simulink model "Integration"  (R2024b)
settings: Solver=VariableStepAuto  StartTime=0.0  StopTime=4  RelTol=1e-3
undefined symbols (not defined in the file): Ion, Lithium, Ts_Control
libraries: spsSeriesRLCBranchLib x37, ee_lib x30, nesl_utility x30, spsCurrentVoltageSimscapeInterfaceLib x18, slpidlib x9, spsThreePhaseVIMeasurementLib x7, spsParallelRLCBranchLib x7, spsThreePhaseSeriesRLCBranchLib x7, spsGroundLib x7, spsDiodeLib x6, spsIGBTDiodeLib x6, spsPWMGeneratorDCDCLib x6
(part 1 of 4)
settings Model: Creator=DELL  LastModifiedBy=DELL

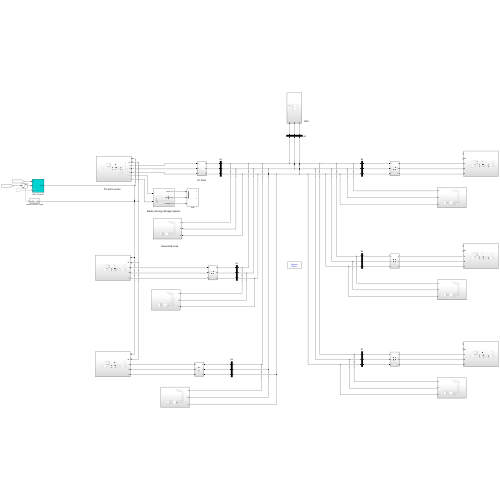
[thumbnail: Simulink's stored preview of the top-level diagram]
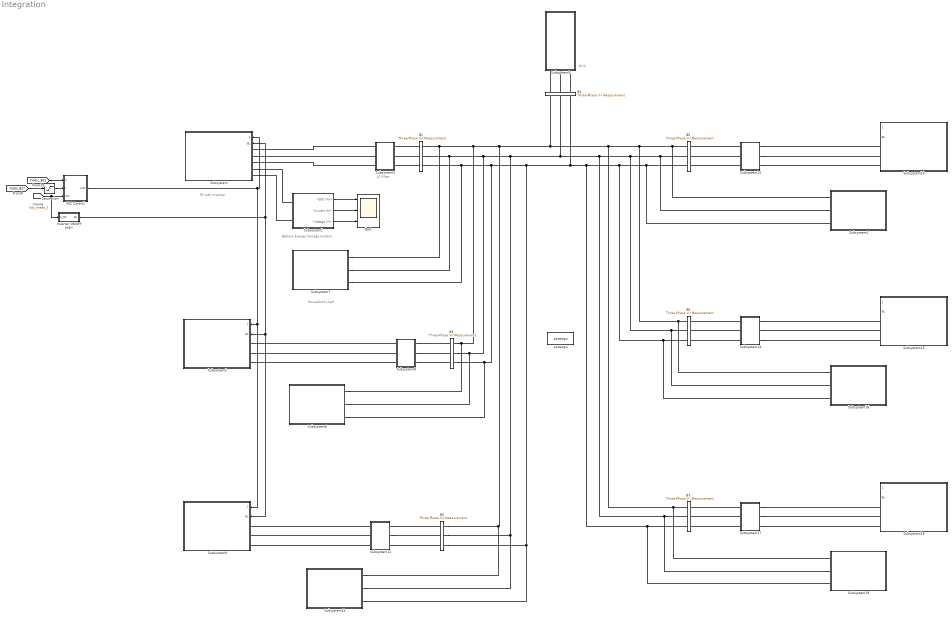
== system Integration ==
  note: Household Load
  note: LC Filter
  note: Battery Energy Storage System
  note: Grid
  note: PV with Inverter
  B1 : spsThreePhaseVIMeasurementLib/Three-Phase V-I Measurement  VoltageMeasurement=phase-to-phase  SetLabelV=on  LabelV=Vabc_B1  Vpu=off  VpuLL=off  CurrentMeasurement=yes  SetLabelI=on  LabelI=Iabc_B1  Ipu=off  Pbase=100e6  Vbase=1000  OutputType=Magnitude  PhasorSimulation=off  PSBequivalent=0
  B2 : spsThreePhaseVIMeasurementLib/Three-Phase V-I Measurement  VoltageMeasurement=phase-to-phase  SetLabelV=on  LabelV=Vabc_B2  Vpu=off  VpuLL=off  CurrentMeasurement=yes  SetLabelI=on  LabelI=Iabc_B2  Ipu=off  Pbase=100e6  Vbase=500e3  OutputType=Magnitude  PhasorSimulation=off  PSBequivalent=0
  B3 : spsThreePhaseVIMeasurementLib/Three-Phase V-I Measurement  VoltageMeasurement=phase-to-phase  SetLabelV=on  LabelV=Vabc_B3  Vpu=off  VpuLL=off  CurrentMeasurement=yes  SetLabelI=on  LabelI=Iabc_B3  Ipu=off  Pbase=100e6  Vbase=1000  OutputType=Magnitude  PhasorSimulation=off  PSBequivalent=0
  B4 : spsThreePhaseVIMeasurementLib/Three-Phase V-I Measurement  VoltageMeasurement=phase-to-phase  SetLabelV=on  LabelV=Vabc_B4  Vpu=off  VpuLL=off  CurrentMeasurement=yes  SetLabelI=on  LabelI=Iabc_B4  Ipu=off  Pbase=100e6  Vbase=1000  OutputType=Magnitude  PhasorSimulation=off  PSBequivalent=0
  B5 : spsThreePhaseVIMeasurementLib/Three-Phase V-I Measurement  VoltageMeasurement=phase-to-phase  SetLabelV=on  LabelV=Vabc_B5  Vpu=off  VpuLL=off  CurrentMeasurement=yes  SetLabelI=on  LabelI=Iabc_B5  Ipu=off  Pbase=100e6  Vbase=1000  OutputType=Magnitude  PhasorSimulation=off  PSBequivalent=0
  B6 : spsThreePhaseVIMeasurementLib/Three-Phase V-I Measurement  VoltageMeasurement=phase-to-phase  SetLabelV=on  LabelV=Vabc_B6  Vpu=off  VpuLL=off  CurrentMeasurement=yes  SetLabelI=on  LabelI=Iabc_B6  Ipu=off  Pbase=100e6  Vbase=1000  OutputType=Magnitude  PhasorSimulation=off  PSBequivalent=0
  B7 : spsThreePhaseVIMeasurementLib/Three-Phase V-I Measurement  VoltageMeasurement=phase-to-phase  SetLabelV=on  LabelV=Vabc_B7  Vpu=off  VpuLL=off  CurrentMeasurement=yes  SetLabelI=on  LabelI=Iabc_B7  Ipu=off  Pbase=100e6  Vbase=1000  OutputType=Magnitude  PhasorSimulation=off  PSBequivalent=0
  Batt : Scope  NumInputPorts=3
  Inverter ON/OFF Logic : Subsystem
  Saturation : Saturate  UpperLimit=40  LowerLimit=-40
  Subsystem : Subsystem
  Subsystem1 : Subsystem
  Subsystem10 : Subsystem
  Subsystem11 : Subsystem
  Subsystem12 : Subsystem
  Subsystem13 : Subsystem
  Subsystem14 : Subsystem
  Subsystem15 : Subsystem
  Subsystem16 : Subsystem
  Subsystem17 : Subsystem
  Subsystem18 : Subsystem
  Subsystem19 : Subsystem
  Subsystem2 : Subsystem
  Subsystem3 : Subsystem
  Subsystem4 : Subsystem
  Subsystem5 : Subsystem
  Subsystem6 : Subsystem
  Subsystem7 : Subsystem
  Subsystem8 : Subsystem
  Subsystem9 : Subsystem
  VSC Control : Subsystem  mask(VSC Main Controller){nom=[ 20e3  50 ], Vnom=[ 400 400 ], Vnom_dc=700, RLxfo=[0  0 ], RLchoke=[0  0  ], K_VDCreg=[18  600], K_Ireg=[0.2 20], Ts=Ts_Control}
      mask prompts: nom "Nominal power and frequency [ Pnom(VA)  Fnom(Hz) ]:"; Vnom "Nominal primary and secondary voltages (Vrms LL) [ Vnom_prim   Vnom_sec ]:"; Vnom_dc "Nominal DC bus voltage (V):"; RLxfo "Total transformer leakage impedance (pu/Pnom) [ Rxfo  Lxf ]"; RLchoke "Choke impedance [ R(ohm) L(H) ]"; K_VDCreg "VDC regultator gains [ Kp  Ki ]:"; K_Ireg "Current regulator gains [ Kp  Ki ]:"; Ts "Sample time"
      mask init:
      | Pnom=nom(1);
      | Fnom=nom(2);
      | Vnom_prim=Vnom(1);
      | Vnom_sec=Vnom(2);
      | Zbase=Vnom_sec^2/Pnom;
      | Rtot_pu=RLxfo(1) + RLchoke(1)/Zbase;
      | Ltot_pu=RLxfo(2) + RLchoke(2)/(Zbase/(2*pi*Fnom));
      | Kp_VDCreg=K_VDCreg(1);
      | Ki_VDCreg=K_VDCreg(2);
      | Kp_Ireg=K_Ireg(1);
      | Ki_Ireg=K_Ireg(2);
      | Vdc_ref=Vnom_dc;
  powergui : spspowerguiLib/powergui  Priority=1  SimulationMode=Discrete  SampleTime=1e-4  frequency=60  Iterations=50  frequencyindice=0  Pbase=100e6  ErrMax=1e-4  UnitsV=kV  UnitsW=MW  buscounter=0  FunctionMessages=off  echomessages=off  EnableUseOfTLC=off  CurrentSourceSwitches=off  DisableSnubberDevices=off  DisableRonSwitches=off  DisableVfSwitches=off  DisplayEquations=off  AutomaticDiscreteSolvers=off  SolverType=Tustin/Backward Euler (TBE)  Interpol=off  ExternalGateDelay=off  methode=off  Ts=100  x0status=blocks  SPID=on  SwTol=0  HookPort=off  NonlinearTolerance=1e-4  nMaxIteration=100  ContinueOnMaxIteration=off  RestoreLinks=warning  ResistiveCurrentMeasurement=off  Frange=[0:2:500]  Ylog=off  Xlog=on  ShowGrid=off  save=off  variable=ZData  structure=0  ZoomFFT=off  StartTime=0.0  cycles=1  DisplayStyle=1  fundamental=60  FreqAxis=off  MaxFrequency=1000  frequencyindicesteady=1  RmsSteady=1  display=off
  wires:
  [Vdc_meas_1] -> Inverter ON/OFF Logic/1(V_DC), VSC Control/3(Vdc)
  [Vabc_B2] -> VSC Control/1(V)
  Saturation/1 -> VSC Control/2(I)
  [Iabc_B2] -> Saturation/1
  Inverter ON/OFF Logic/1(BL) -> Subsystem9/2(BL), Subsystem2/2(BL), Subsystem/2(BL)
  VSC Control/1(Uref) -> Subsystem9/1("  "), Subsystem2/1("  "), Subsystem/1("  ")
  Subsystem1/1(<SOC (%)>) -> Batt/1
  Subsystem1/2(<Current (A)>) -> Batt/2
  Subsystem1/3(<Voltage (V)>) -> Batt/3
  connections:
  B1/RConn1 -- Subsystem7/LConn1 -- Subsystem6/LConn1 -- B3/RConn1 -- Subsystem11/LConn1 -- B4/RConn1 -- Subsystem19/LConn1 -- B7/RConn1 -- Subsystem16/LConn1 -- B6/RConn1 -- Subsystem4/LConn1 -- B5/RConn1 -- B2/RConn1
  B2/RConn3 -- Subsystem11/LConn3 -- B4/RConn3 -- Subsystem6/LConn3 -- B3/RConn3 -- Subsystem7/LConn3 -- B1/RConn3 -- Subsystem19/LConn3 -- B7/RConn3 -- Subsystem16/LConn3 -- B6/RConn3 -- Subsystem4/LConn3 -- B5/RConn3
  B1/RConn2 -- Subsystem7/LConn2 -- Subsystem6/LConn2 -- B3/RConn2 -- Subsystem11/LConn2 -- B4/RConn2 -- Subsystem19/LConn2 -- B7/RConn2 -- Subsystem16/LConn2 -- B6/RConn2 -- Subsystem4/LConn2 -- B5/RConn2 -- B2/RConn2
  B1/LConn3 -- Subsystem3/RConn3
  B1/LConn1 -- Subsystem3/RConn1
  B1/LConn2 -- Subsystem3/RConn2
  Subsystem3/LConn1 -- Subsystem/LConn1
  Subsystem3/LConn2 -- Subsystem/LConn2
  Subsystem3/LConn3 -- Subsystem/LConn3
  B2/LConn1 -- Subsystem5/LConn1
  B2/LConn2 -- Subsystem5/LConn2
  B2/LConn3 -- Subsystem5/LConn3
  Subsystem1/LConn1 -- Subsystem/LConn4
  Subsystem1/LConn2 -- Subsystem/LConn5
  Subsystem8/LConn1 -- Subsystem2/LConn1
  Subsystem8/LConn2 -- Subsystem2/LConn2
  Subsystem8/LConn3 -- Subsystem2/LConn3
  Subsystem8/RConn1 -- B3/LConn1
  Subsystem8/RConn2 -- B3/LConn2
  Subsystem8/RConn3 -- B3/LConn3
  Subsystem12/RConn1 -- B4/LConn1
  Subsystem12/LConn2 -- Subsystem9/LConn2
  Subsystem12/RConn3 -- B4/LConn3
  Subsystem12/LConn3 -- Subsystem9/LConn3
  Subsystem12/LConn1 -- Subsystem9/LConn1
  Subsystem12/RConn2 -- B4/LConn2
  Subsystem10/LConn1 -- Subsystem13/LConn1
  Subsystem10/RConn3 -- B5/LConn3
  Subsystem10/RConn1 -- B5/LConn1
  Subsystem10/LConn3 -- Subsystem13/LConn3
  Subsystem10/LConn2 -- Subsystem13/LConn2
  Subsystem10/RConn2 -- B5/LConn2
  Subsystem14/LConn2 -- Subsystem15/LConn2
  Subsystem14/RConn3 -- B6/LConn3
  Subsystem14/LConn1 -- Subsystem15/LConn1
  Subsystem14/LConn3 -- Subsystem15/LConn3
  Subsystem14/RConn1 -- B6/LConn1
  Subsystem14/RConn2 -- B6/LConn2
  Subsystem17/LConn2 -- Subsystem18/LConn2
  Subsystem17/RConn3 -- B7/LConn3
  Subsystem17/LConn1 -- Subsystem18/LConn1
  Subsystem17/LConn3 -- Subsystem18/LConn3
  Subsystem17/RConn1 -- B7/LConn1
  Subsystem17/RConn2 -- B7/LConn2

== system Integration/Inverter ON//OFF Logic ==
  V_DC : Inport
  AND : Logic  Operator=NAND  IconShape=distinctive  AllPortsSameDT=off  OutDataTypeStr=boolean
  Compare To Constant : simulink/Logic and Bit Operations/Compare To Constant  relop=>=  const=200  OutDataTypeStr=boolean
  Constant : Constant
  Data Type Conversion : DataTypeConversion  OutDataTypeStr=double  SaturateOnIntegerOverflow=off  RndMeth=Floor
  BL : Outport
  tag scope: inv_cont_1=global
  wires:
  Data Type Conversion/1 -> [inv_cont_1], BL/1
  V_DC/1 -> Compare To Constant/1
  AND/1 -> Data Type Conversion/1
  Compare To Constant/1 -> AND/1
  Constant/1 -> AND/2

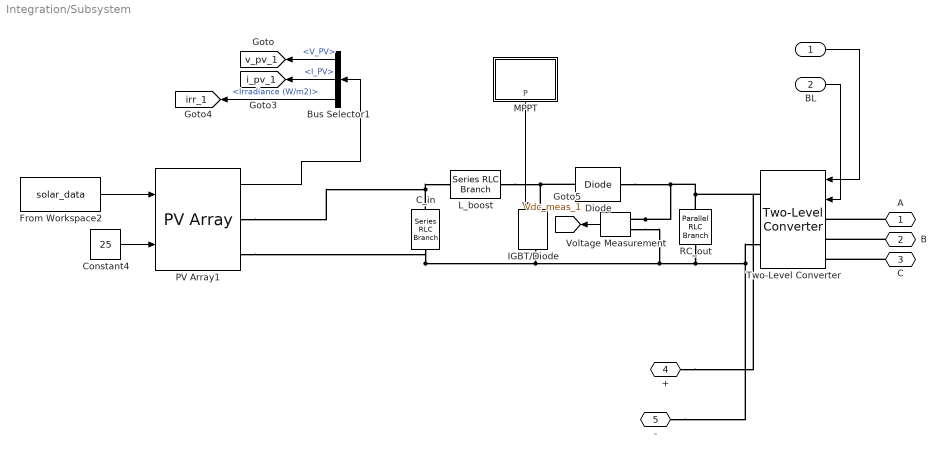
== system Integration/Subsystem ==
  "  " : Inport
  BL : Inport  Port=2
  Bus Selector1 : BusSelector  OutputSignals=V_PV,I_PV,Irradiance (W/m2)
  C_in : spsSeriesRLCBranchLib/Series RLC Branch  LConnTagsString=__new0  RConnTagsString=__new0  BranchType=C  Resistance=1e-5  Inductance=1e-3  SetiL0=off  InitialCurrent=0  Capacitance=850e-6  Setx0=off  InitialVoltage=426.5  Measurements=Branch voltage and current
  Constant4 : Constant  Value=25
  Diode : spsDiodeLib/Diode  Ron=0.001  Lon=0  Vf=0.8  IC=0  UseSnubber=0  Rs=500  Cs=250e-9  Measurements=off
  From Workspace2 : FromWorkspace  VariableName=solar_data  OutDataTypeStr=double  SampleTime=0.01
  IGBT/Diode : spsIGBTDiodeLib/IGBT//Diode  Ron=1e-3  Rs=1e5  Cs=inf  Measurements=off
  L_boost : spsSeriesRLCBranchLib/Series RLC Branch  LConnTagsString=__new0  RConnTagsString=__new0  BranchType=L  Resistance=1e-3  Inductance=36e-3  SetiL0=off  InitialCurrent=0  Capacitance=100e-6  Setx0=off  InitialVoltage=230  Measurements=None
  MPPT : Subsystem
  PV Array1 : spsPVArrayLib/PV Array  Npar=8  Nser=5  PlotType=array @ 1000 W/m2 & specified temperatures  S_vec="[ 1000  500  100 ]"  Temp_C_vec="[ 45 25  ]"  ModuleName=SunPower SPR-415E-WHT-D  PlotWhenSelected=off  Pm=414.801  Ncell=128  Voc=85.3  Isc=6.09  Vm=72.9  Im=5.69  beta_Voc_pc=-0.229  alpha_Isc_pc=0.030706  beta_Voc=-0.19534  alpha_Isc=0.00187  IL=6.0978  I0=7.1698e-13  nI=0.87223  Rsh=419.7781  Rs=0.53711  RobustModel=off  RobustCellTemperature=313.3991  BAL=on  Tc=1e-6  Tfilter=5e-5
  RC_out : spsParallelRLCBranchLib/Parallel RLC Branch  LConnTagsString=a  RConnTagsString=__new0  BranchType=C  Resistance=5  Inductance=1e-3  SetiL0=off  InitialCurrent=0  Capacitance=5*636e-6  Setx0=off  InitialVoltage=700  Measurements=None
  Two-Level Converter : spsTwoLevelConverterLib/Two-Level Converter  ModelType=Switching devices  Ron=1e-3  Rs=1e6  Cs=inf  Vforward=[0,0]  Ron_Diode=1e-3  Rs_Diode=1e6  Cs_Diode=inf  Vf_Diode=1e-3  Rs_CurrentSource=inf  Ron_ACsource=1e-3
      settings: LibrarySourceBlock=sps_lib/Power Electronics/Two-Level Converter
  Voltage Measurement : spsVoltageMeasurementLib/Voltage Measurement  PhasorSimulation=off  OutputType=Complex  PSBequivalent=0
  A : PMIOPort  Side=Left
  B : PMIOPort  Port=2  Side=Left
  C : PMIOPort  Port=3  Side=Left
  + : PMIOPort  Port=4  Side=Left
  - : PMIOPort  Port=5  Side=Left
  tag scope: Vdc_meas_1=global, i_pv_1=global, irr_1=global, v_pv_1=global
  wires:
  Voltage Measurement/1 -> [Vdc_meas_1]
  BL/1 -> Two-Level Converter/2
  Bus Selector1/3 -> [irr_1]  "<Irradiance (W/m2)>"
  Bus Selector1/1 -> [v_pv_1]  "<V_PV>"
  Constant4/1 -> PV Array1/2
  "  "/1 -> Two-Level Converter/1
  Bus Selector1/2 -> [i_pv_1]  "<I_PV>"
  PV Array1/1 -> Bus Selector1/1
  MPPT/1(P) -> IGBT/Diode/1
  From Workspace2/1 -> PV Array1/1
  connections:
  A/RConn1 -- Two-Level Converter/LConn1
  PV Array1/RConn2 -- C_in/RConn1 -- IGBT/Diode/RConn1 -- Voltage Measurement/LConn2 -- RC_out/RConn1 -- -/RConn1 -- Two-Level Converter/RConn2
  IGBT/Diode/LConn1 -- L_boost/RConn1 -- Diode/LConn1
  PV Array1/RConn1 -- L_boost/LConn1 -- C_in/LConn1
  Voltage Measurement/LConn1 -- +/RConn1 -- Two-Level Converter/RConn1 -- RC_out/LConn1 -- Diode/RConn1
  C/RConn1 -- Two-Level Converter/LConn3
  B/RConn1 -- Two-Level Converter/LConn2

== system Integration/Subsystem1 ==
  BATT chg-dshg logic : Subsystem
  Battery : spsBatteryLib/Battery  BatType=Lithium-Ion  NomV=24  NomQ=20  SOC=0  Batt_Tr=0.01  PresetModel=on  MaxQ=20  MinV=18  FullV=27.9357  Dis_rate=8.6957  R=0.012  Normal_OP=18.087  expZone="[25.9293     0.982609]"
  Bus Selector : BusSelector  OutputSignals=SOC (%),Current (A),Voltage (V)
  L_B : spsSeriesRLCBranchLib/Series RLC Branch  LConnTagsString=__new0  RConnTagsString=__new0  BranchType=L  Resistance=1e-3  Inductance=1e-3  SetiL0=off  InitialCurrent=0  Capacitance=100e-6  Setx0=off  InitialVoltage=230  Measurements=None
  RC_B : spsParallelRLCBranchLib/Parallel RLC Branch  LConnTagsString=a  RConnTagsString=__new0  BranchType=C  Resistance=5  Inductance=1e-3  SetiL0=off  InitialCurrent=0  Capacitance=50e-6  Setx0=off  InitialVoltage=700  Measurements=None
  Two-Quadrant DC/DC Converter : spsTwoQuadrantDCDCConverterLib/Two-Quadrant DC//DC Converter  ModelType=Average model (D-controlled)  Ron=1e-3  Rs=1e6  Cs=inf  Vforward=[0,0]  Ron_Diode=1e-3  Rs_Diode=1e6  Cs_Diode=inf  Vf_Diode=1e-3  Rs_CurrentSource=inf  Ron_ACsource=1e-3
  + : PMIOPort  Side=Left
  - : PMIOPort  Port=2  Side=Left
  <SOC (%)> : Outport
  <Current (A)> : Outport  Port=2
  <Voltage (V)> : Outport  Port=3
  wires:
  Battery/1 -> Bus Selector/1
  BATT chg-dshg logic/2(BL) -> Two-Quadrant DC/DC Converter/2
  Bus Selector/3 -> <Voltage (V)>/1, BATT chg-dshg logic/2(V_batt)  "<Voltage (V)>"
  Bus Selector/1 -> <SOC (%)>/1, BATT chg-dshg logic/1(SoC)  "<SOC (%)>"
  BATT chg-dshg logic/1(D) -> Two-Quadrant DC/DC Converter/1
  Bus Selector/2 -> <Current (A)>/1  "<Current (A)>"
  connections:
  RC_B/LConn1 -- +/RConn1 -- Two-Quadrant DC/DC Converter/RConn1
  L_B/LConn1 -- Battery/LConn1
  Battery/LConn2 -- -/RConn1 -- RC_B/RConn1 -- Two-Quadrant DC/DC Converter/RConn2
  L_B/RConn1 -- Two-Quadrant DC/DC Converter/LConn1

== system Integration/Subsystem10 ==
  Series RLC Branch1 : spsSeriesRLCBranchLib/Series RLC Branch  LConnTagsString=__new0  RConnTagsString=__new0  BranchType=RC  Resistance=10  Inductance=1e-3  SetiL0=off  InitialCurrent=0  Capacitance=3*15e-6  Setx0=off  InitialVoltage=0  Measurements=None
  Series RLC Branch2 : spsSeriesRLCBranchLib/Series RLC Branch  LConnTagsString=__new0  RConnTagsString=__new0  BranchType=RC  Resistance=10  Inductance=1e-3  SetiL0=off  InitialCurrent=0  Capacitance=3*15e-6  Setx0=off  InitialVoltage=0  Measurements=None
  Series RLC Branch3 : spsSeriesRLCBranchLib/Series RLC Branch  LConnTagsString=__new0  RConnTagsString=__new0  BranchType=RC  Resistance=10  Inductance=1e-3  SetiL0=off  InitialCurrent=0  Capacitance=3*15e-6  Setx0=off  InitialVoltage=0  Measurements=None
  Three-Phase Series RLC Branch1 : spsThreePhaseSeriesRLCBranchLib/Three-Phase Series RLC Branch  LConnTagsString=A|B|C  RConnTagsString=A|B|C  BranchType=L  Resistance=1  Inductance=3*6e-3  Capacitance=1e-6  Measurements=None
  Three-Phase Breaker : spsThreePhaseBreakerLib/Three-Phase Breaker  InitialState=closed  SwitchA=on  SwitchB=on  SwitchC=on  SwitchTimes="[1/60  5/60]"  External=off  BreakerResistance=0.01  SnubberResistance=1e6  SnubberCapacitance=inf  Measurements=None
  A : PMIOPort  Side=Left
  B : PMIOPort  Port=2  Side=Left
  C : PMIOPort  Port=3  Side=Left
  a : PMIOPort  Port=4  Side=Right
  b : PMIOPort  Port=5  Side=Right
  c : PMIOPort  Port=6  Side=Right
  connections:
  Series RLC Branch1/LConn1 -- Three-Phase Series RLC Branch1/RConn2 -- Three-Phase Breaker/LConn2 -- Series RLC Branch3/RConn1
  Series RLC Branch1/RConn1 -- Three-Phase Breaker/LConn3 -- Three-Phase Series RLC Branch1/RConn3 -- Series RLC Branch2/RConn1
  Series RLC Branch3/LConn1 -- Three-Phase Series RLC Branch1/RConn1 -- Three-Phase Breaker/LConn1 -- Series RLC Branch2/LConn1
  Three-Phase Series RLC Branch1/LConn1 -- A/RConn1
  Three-Phase Series RLC Branch1/LConn2 -- B/RConn1
  Three-Phase Series RLC Branch1/LConn3 -- C/RConn1
  Three-Phase Breaker/RConn1 -- a/RConn1
  b/RConn1 -- Three-Phase Breaker/RConn2
  c/RConn1 -- Three-Phase Breaker/RConn3

== system Integration/Subsystem11 ==
  Ground1 : spsGroundLib/Ground  LConnTagsString=a
  Subsystem2 : Subsystem
  load : Scope  NumInputPorts=4
  A : PMIOPort  Side=Left
  B : PMIOPort  Port=2  Side=Left
  C : PMIOPort  Port=3  Side=Left
  wires:
  Subsystem2/4(Q_load) -> load/4
  Subsystem2/2(I_load) -> load/2
  Subsystem2/3(P_load) -> load/3
  Subsystem2/1(V_load) -> load/1
  connections:
  Subsystem2/LConn2 -- B/RConn1
  Subsystem2/LConn4 -- Ground1/LConn1
  Subsystem2/LConn1 -- A/RConn1
  Subsystem2/LConn3 -- C/RConn1

== system Integration/Subsystem12 ==
  Series RLC Branch1 : spsSeriesRLCBranchLib/Series RLC Branch  LConnTagsString=__new0  RConnTagsString=__new0  BranchType=RC  Resistance=10  Inductance=1e-3  SetiL0=off  InitialCurrent=0  Capacitance=3*15e-6  Setx0=off  InitialVoltage=0  Measurements=None
  Series RLC Branch2 : spsSeriesRLCBranchLib/Series RLC Branch  LConnTagsString=__new0  RConnTagsString=__new0  BranchType=RC  Resistance=10  Inductance=1e-3  SetiL0=off  InitialCurrent=0  Capacitance=3*15e-6  Setx0=off  InitialVoltage=0  Measurements=None
  Series RLC Branch3 : spsSeriesRLCBranchLib/Series RLC Branch  LConnTagsString=__new0  RConnTagsString=__new0  BranchType=RC  Resistance=10  Inductance=1e-3  SetiL0=off  InitialCurrent=0  Capacitance=3*15e-6  Setx0=off  InitialVoltage=0  Measurements=None
  Three-Phase Series RLC Branch1 : spsThreePhaseSeriesRLCBranchLib/Three-Phase Series RLC Branch  LConnTagsString=A|B|C  RConnTagsString=A|B|C  BranchType=L  Resistance=1  Inductance=3*6e-3  Capacitance=1e-6  Measurements=None
  Three-Phase Breaker : spsThreePhaseBreakerLib/Three-Phase Breaker  InitialState=closed  SwitchA=on  SwitchB=on  SwitchC=on  SwitchTimes="[1/60  5/60]"  External=off  BreakerResistance=0.01  SnubberResistance=1e6  SnubberCapacitance=inf  Measurements=None
  A : PMIOPort  Side=Left
  B : PMIOPort  Port=2  Side=Left
  C : PMIOPort  Port=3  Side=Left
  a : PMIOPort  Port=4  Side=Right
  b : PMIOPort  Port=5  Side=Right
  c : PMIOPort  Port=6  Side=Right
  connections:
  Series RLC Branch1/LConn1 -- Three-Phase Series RLC Branch1/RConn2 -- Three-Phase Breaker/LConn2 -- Series RLC Branch3/RConn1
  Series RLC Branch1/RConn1 -- Three-Phase Breaker/LConn3 -- Three-Phase Series RLC Branch1/RConn3 -- Series RLC Branch2/RConn1
  Series RLC Branch3/LConn1 -- Three-Phase Series RLC Branch1/RConn1 -- Three-Phase Breaker/LConn1 -- Series RLC Branch2/LConn1
  Three-Phase Series RLC Branch1/LConn1 -- A/RConn1
  Three-Phase Series RLC Branch1/LConn2 -- B/RConn1
  Three-Phase Series RLC Branch1/LConn3 -- C/RConn1
  Three-Phase Breaker/RConn1 -- a/RConn1
  b/RConn1 -- Three-Phase Breaker/RConn2
  c/RConn1 -- Three-Phase Breaker/RConn3

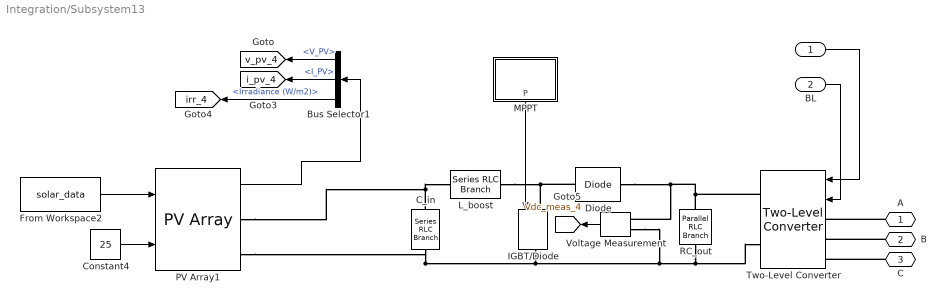
== system Integration/Subsystem13 ==
  "  " : Inport
  BL : Inport  Port=2
  Bus Selector1 : BusSelector  OutputSignals=V_PV,I_PV,Irradiance (W/m2)
  C_in : spsSeriesRLCBranchLib/Series RLC Branch  LConnTagsString=__new0  RConnTagsString=__new0  BranchType=C  Resistance=1e-5  Inductance=1e-3  SetiL0=off  InitialCurrent=0  Capacitance=1200e-6  Setx0=off  InitialVoltage=426.5  Measurements=Branch voltage and current
  Constant4 : Constant  Value=25
  Diode : spsDiodeLib/Diode  Ron=0.001  Lon=0  Vf=0.8  IC=0  UseSnubber=0  Rs=500  Cs=250e-9  Measurements=off
  From Workspace2 : FromWorkspace  VariableName=solar_data  OutDataTypeStr=double  SampleTime=0.01
  IGBT/Diode : spsIGBTDiodeLib/IGBT//Diode  Ron=1e-3  Rs=1e5  Cs=inf  Measurements=off
  L_boost : spsSeriesRLCBranchLib/Series RLC Branch  LConnTagsString=__new0  RConnTagsString=__new0  BranchType=L  Resistance=1e-3  Inductance=70e-3  SetiL0=off  InitialCurrent=0  Capacitance=100e-6  Setx0=off  InitialVoltage=230  Measurements=None
  MPPT : Subsystem
  PV Array1 : spsPVArrayLib/PV Array  Npar=7  Nser=4  PlotType=array @ 1000 W/m2 & specified temperatures  S_vec="[ 1000  500  100 ]"  Temp_C_vec="[ 45 25  ]"  ModuleName=SunPower SPR-415E-WHT-D  PlotWhenSelected=off  Pm=414.801  Ncell=128  Voc=85.3  Isc=6.09  Vm=72.9  Im=5.69  beta_Voc_pc=-0.229  alpha_Isc_pc=0.030706  beta_Voc=-0.19534  alpha_Isc=0.00187  IL=6.0978  I0=7.1698e-13  nI=0.87223  Rsh=419.7781  Rs=0.53711  RobustModel=off  RobustCellTemperature=313.3991  BAL=on  Tc=1e-6  Tfilter=5e-5
  RC_out : spsParallelRLCBranchLib/Parallel RLC Branch  LConnTagsString=a  RConnTagsString=__new0  BranchType=C  Resistance=5  Inductance=1e-3  SetiL0=off  InitialCurrent=0  Capacitance=5*730e-6  Setx0=off  InitialVoltage=700  Measurements=None
  Two-Level Converter : spsTwoLevelConverterLib/Two-Level Converter  ModelType=Switching devices  Ron=1e-3  Rs=1e6  Cs=inf  Vforward=[0,0]  Ron_Diode=1e-3  Rs_Diode=1e6  Cs_Diode=inf  Vf_Diode=1e-3  Rs_CurrentSource=inf  Ron_ACsource=1e-3
  Voltage Measurement : spsVoltageMeasurementLib/Voltage Measurement  PhasorSimulation=off  OutputType=Complex  PSBequivalent=0
  A : PMIOPort  Side=Left
  B : PMIOPort  Port=2  Side=Left
  C : PMIOPort  Port=3  Side=Left
  tag scope: Vdc_meas_4=global, i_pv_4=global, irr_4=global, v_pv_4=global
  wires:
  Voltage Measurement/1 -> [Vdc_meas_4]
  BL/1 -> Two-Level Converter/2
  Bus Selector1/3 -> [irr_4]  "<Irradiance (W/m2)>"
  Bus Selector1/1 -> [v_pv_4]  "<V_PV>"
  Constant4/1 -> PV Array1/2
  "  "/1 -> Two-Level Converter/1
  Bus Selector1/2 -> [i_pv_4]  "<I_PV>"
  PV Array1/1 -> Bus Selector1/1
  MPPT/1(P) -> IGBT/Diode/1
  From Workspace2/1 -> PV Array1/1
  connections:
  A/RConn1 -- Two-Level Converter/LConn1
  Two-Level Converter/RConn2 -- RC_out/RConn1 -- Voltage Measurement/LConn2 -- IGBT/Diode/RConn1 -- C_in/RConn1 -- PV Array1/RConn2
  Diode/LConn1 -- IGBT/Diode/LConn1 -- L_boost/RConn1
  C_in/LConn1 -- PV Array1/RConn1 -- L_boost/LConn1
  RC_out/LConn1 -- Diode/RConn1 -- Voltage Measurement/LConn1 -- Two-Level Converter/RConn1
  C/RConn1 -- Two-Level Converter/LConn3
  B/RConn1 -- Two-Level Converter/LConn2

== system Integration/Subsystem14 ==
  Series RLC Branch1 : spsSeriesRLCBranchLib/Series RLC Branch  LConnTagsString=__new0  RConnTagsString=__new0  BranchType=RC  Resistance=10  Inductance=1e-3  SetiL0=off  InitialCurrent=0  Capacitance=3*15e-6  Setx0=off  InitialVoltage=0  Measurements=None
  Series RLC Branch2 : spsSeriesRLCBranchLib/Series RLC Branch  LConnTagsString=__new0  RConnTagsString=__new0  BranchType=RC  Resistance=10  Inductance=1e-3  SetiL0=off  InitialCurrent=0  Capacitance=3*15e-6  Setx0=off  InitialVoltage=0  Measurements=None
  Series RLC Branch3 : spsSeriesRLCBranchLib/Series RLC Branch  LConnTagsString=__new0  RConnTagsString=__new0  BranchType=RC  Resistance=10  Inductance=1e-3  SetiL0=off  InitialCurrent=0  Capacitance=3*15e-6  Setx0=off  InitialVoltage=0  Measurements=None
  Three-Phase Series RLC Branch1 : spsThreePhaseSeriesRLCBranchLib/Three-Phase Series RLC Branch  LConnTagsString=A|B|C  RConnTagsString=A|B|C  BranchType=L  Resistance=1  Inductance=3*6e-3  Capacitance=1e-6  Measurements=None
  Three-Phase Breaker : spsThreePhaseBreakerLib/Three-Phase Breaker  InitialState=closed  SwitchA=on  SwitchB=on  SwitchC=on  SwitchTimes="[1/60  5/60]"  External=off  BreakerResistance=0.01  SnubberResistance=1e6  SnubberCapacitance=inf  Measurements=None
  A : PMIOPort  Side=Left
  B : PMIOPort  Port=2  Side=Left
  C : PMIOPort  Port=3  Side=Left
  a : PMIOPort  Port=4  Side=Right
  b : PMIOPort  Port=5  Side=Right
  c : PMIOPort  Port=6  Side=Right
  connections:
  Series RLC Branch1/LConn1 -- Three-Phase Series RLC Branch1/RConn2 -- Three-Phase Breaker/LConn2 -- Series RLC Branch3/RConn1
  Series RLC Branch1/RConn1 -- Three-Phase Breaker/LConn3 -- Three-Phase Series RLC Branch1/RConn3 -- Series RLC Branch2/RConn1
  Series RLC Branch3/LConn1 -- Three-Phase Series RLC Branch1/RConn1 -- Three-Phase Breaker/LConn1 -- Series RLC Branch2/LConn1
  Three-Phase Series RLC Branch1/LConn1 -- A/RConn1
  Three-Phase Series RLC Branch1/LConn2 -- B/RConn1
  Three-Phase Series RLC Branch1/LConn3 -- C/RConn1
  Three-Phase Breaker/RConn1 -- a/RConn1
  b/RConn1 -- Three-Phase Breaker/RConn2
  c/RConn1 -- Three-Phase Breaker/RConn3

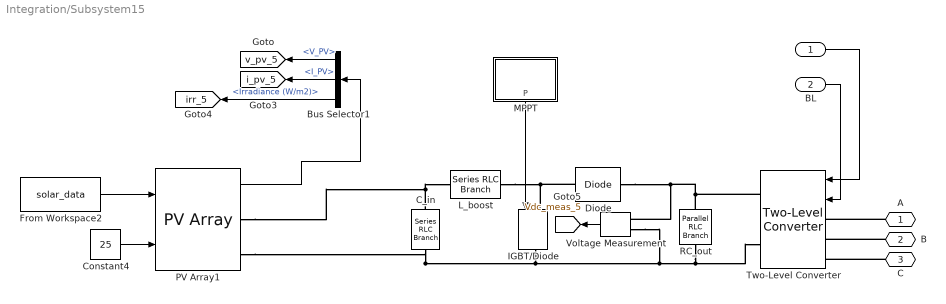
== system Integration/Subsystem15 ==
  "  " : Inport
  BL : Inport  Port=2
  Bus Selector1 : BusSelector  OutputSignals=V_PV,I_PV,Irradiance (W/m2)
  C_in : spsSeriesRLCBranchLib/Series RLC Branch  LConnTagsString=__new0  RConnTagsString=__new0  BranchType=C  Resistance=1e-5  Inductance=1e-3  SetiL0=off  InitialCurrent=0  Capacitance=1696e-6  Setx0=off  InitialVoltage=426.5  Measurements=Branch voltage and current
  Constant4 : Constant  Value=25
  Diode : spsDiodeLib/Diode  Ron=0.001  Lon=0  Vf=0.8  IC=0  UseSnubber=0  Rs=500  Cs=250e-9  Measurements=off
  From Workspace2 : FromWorkspace  VariableName=solar_data  OutDataTypeStr=double  SampleTime=0.01
  IGBT/Diode : spsIGBTDiodeLib/IGBT//Diode  Ron=1e-3  Rs=1e5  Cs=inf  Measurements=off
  L_boost : spsSeriesRLCBranchLib/Series RLC Branch  LConnTagsString=__new0  RConnTagsString=__new0  BranchType=L  Resistance=1e-3  Inductance=76e-3  SetiL0=off  InitialCurrent=0  Capacitance=100e-6  Setx0=off  InitialVoltage=230  Measurements=None
  MPPT : Subsystem
  PV Array1 : spsPVArrayLib/PV Array  Npar=6  Nser=3  PlotType=array @ 1000 W/m2 & specified temperatures  S_vec="[ 1000  500  100 ]"  Temp_C_vec="[ 45 25  ]"  ModuleName=SunPower SPR-415E-WHT-D  PlotWhenSelected=off  Pm=414.801  Ncell=128  Voc=85.3  Isc=6.09  Vm=72.9  Im=5.69  beta_Voc_pc=-0.229  alpha_Isc_pc=0.030706  beta_Voc=-0.19534  alpha_Isc=0.00187  IL=6.0978  I0=7.1698e-13  nI=0.87223  Rsh=419.7781  Rs=0.53711  RobustModel=off  RobustCellTemperature=313.3991  BAL=on  Tc=1e-6  Tfilter=5e-5
  RC_out : spsParallelRLCBranchLib/Parallel RLC Branch  LConnTagsString=a  RConnTagsString=__new0  BranchType=C  Resistance=5  Inductance=1e-3  SetiL0=off  InitialCurrent=0  Capacitance=5*774e-6  Setx0=off  InitialVoltage=700  Measurements=None
  Two-Level Converter : spsTwoLevelConverterLib/Two-Level Converter  ModelType=Switching devices  Ron=1e-3  Rs=1e6  Cs=inf  Vforward=[0,0]  Ron_Diode=1e-3  Rs_Diode=1e6  Cs_Diode=inf  Vf_Diode=1e-3  Rs_CurrentSource=inf  Ron_ACsource=1e-3
  Voltage Measurement : spsVoltageMeasurementLib/Voltage Measurement  PhasorSimulation=off  OutputType=Complex  PSBequivalent=0
  A : PMIOPort  Side=Left
  B : PMIOPort  Port=2  Side=Left
  C : PMIOPort  Port=3  Side=Left
  tag scope: Vdc_meas_5=global, i_pv_5=global, irr_5=global, v_pv_5=global
  wires:
  Voltage Measurement/1 -> [Vdc_meas_5]
  BL/1 -> Two-Level Converter/2
  Bus Selector1/3 -> [irr_5]  "<Irradiance (W/m2)>"
  Bus Selector1/1 -> [v_pv_5]  "<V_PV>"
  Constant4/1 -> PV Array1/2
  "  "/1 -> Two-Level Converter/1
  Bus Selector1/2 -> [i_pv_5]  "<I_PV>"
  PV Array1/1 -> Bus Selector1/1
  MPPT/1(P) -> IGBT/Diode/1
  From Workspace2/1 -> PV Array1/1
  connections:
  A/RConn1 -- Two-Level Converter/LConn1
  Two-Level Converter/RConn2 -- RC_out/RConn1 -- Voltage Measurement/LConn2 -- IGBT/Diode/RConn1 -- C_in/RConn1 -- PV Array1/RConn2
  Diode/LConn1 -- IGBT/Diode/LConn1 -- L_boost/RConn1
  C_in/LConn1 -- PV Array1/RConn1 -- L_boost/LConn1
  RC_out/LConn1 -- Diode/RConn1 -- Voltage Measurement/LConn1 -- Two-Level Converter/RConn1
  C/RConn1 -- Two-Level Converter/LConn3
  B/RConn1 -- Two-Level Converter/LConn2

== system Integration/Subsystem16 ==
  Ground1 : spsGroundLib/Ground  LConnTagsString=a
  Subsystem2 : Subsystem
  load : Scope  NumInputPorts=4
  A : PMIOPort  Side=Left
  B : PMIOPort  Port=2  Side=Left
  C : PMIOPort  Port=3  Side=Left
  wires:
  Subsystem2/4(Q_load) -> load/4
  Subsystem2/2(I_load) -> load/2
  Subsystem2/3(P_load) -> load/3
  Subsystem2/1(V_load) -> load/1
  connections:
  Subsystem2/LConn2 -- B/RConn1
  Subsystem2/LConn4 -- Ground1/LConn1
  Subsystem2/LConn1 -- A/RConn1
  Subsystem2/LConn3 -- C/RConn1

== system Integration/Subsystem17 ==
  Series RLC Branch1 : spsSeriesRLCBranchLib/Series RLC Branch  LConnTagsString=__new0  RConnTagsString=__new0  BranchType=RC  Resistance=10  Inductance=1e-3  SetiL0=off  InitialCurrent=0  Capacitance=3*15e-6  Setx0=off  InitialVoltage=0  Measurements=None
  Series RLC Branch2 : spsSeriesRLCBranchLib/Series RLC Branch  LConnTagsString=__new0  RConnTagsString=__new0  BranchType=RC  Resistance=10  Inductance=1e-3  SetiL0=off  InitialCurrent=0  Capacitance=3*15e-6  Setx0=off  InitialVoltage=0  Measurements=None
  Series RLC Branch3 : spsSeriesRLCBranchLib/Series RLC Branch  LConnTagsString=__new0  RConnTagsString=__new0  BranchType=RC  Resistance=10  Inductance=1e-3  SetiL0=off  InitialCurrent=0  Capacitance=3*15e-6  Setx0=off  InitialVoltage=0  Measurements=None
  Three-Phase Series RLC Branch1 : spsThreePhaseSeriesRLCBranchLib/Three-Phase Series RLC Branch  LConnTagsString=A|B|C  RConnTagsString=A|B|C  BranchType=L  Resistance=1  Inductance=3*6e-3  Capacitance=1e-6  Measurements=None
  Three-Phase Breaker : spsThreePhaseBreakerLib/Three-Phase Breaker  InitialState=closed  SwitchA=on  SwitchB=on  SwitchC=on  SwitchTimes="[1/60  5/60]"  External=off  BreakerResistance=0.01  SnubberResistance=1e6  SnubberCapacitance=inf  Measurements=None
  A : PMIOPort  Side=Left
  B : PMIOPort  Port=2  Side=Left
  C : PMIOPort  Port=3  Side=Left
  a : PMIOPort  Port=4  Side=Right
  b : PMIOPort  Port=5  Side=Right
  c : PMIOPort  Port=6  Side=Right
  connections:
  Series RLC Branch1/LConn1 -- Three-Phase Series RLC Branch1/RConn2 -- Three-Phase Breaker/LConn2 -- Series RLC Branch3/RConn1
  Series RLC Branch1/RConn1 -- Three-Phase Breaker/LConn3 -- Three-Phase Series RLC Branch1/RConn3 -- Series RLC Branch2/RConn1
  Series RLC Branch3/LConn1 -- Three-Phase Series RLC Branch1/RConn1 -- Three-Phase Breaker/LConn1 -- Series RLC Branch2/LConn1
  Three-Phase Series RLC Branch1/LConn1 -- A/RConn1
  Three-Phase Series RLC Branch1/LConn2 -- B/RConn1
  Three-Phase Series RLC Branch1/LConn3 -- C/RConn1
  Three-Phase Breaker/RConn1 -- a/RConn1
  b/RConn1 -- Three-Phase Breaker/RConn2
  c/RConn1 -- Three-Phase Breaker/RConn3

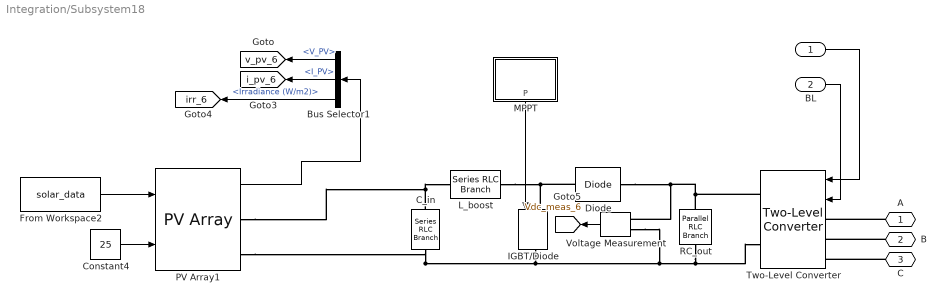
== system Integration/Subsystem18 ==
  "  " : Inport
  BL : Inport  Port=2
  Bus Selector1 : BusSelector  OutputSignals=V_PV,I_PV,Irradiance (W/m2)
  C_in : spsSeriesRLCBranchLib/Series RLC Branch  LConnTagsString=__new0  RConnTagsString=__new0  BranchType=C  Resistance=1e-5  Inductance=1e-3  SetiL0=off  InitialCurrent=0  Capacitance=2525e-6  Setx0=off  InitialVoltage=426.5  Measurements=Branch voltage and current
  Constant4 : Constant  Value=25
  Diode : spsDiodeLib/Diode  Ron=0.001  Lon=0  Vf=0.8  IC=0  UseSnubber=0  Rs=500  Cs=250e-9  Measurements=off
  From Workspace2 : FromWorkspace  VariableName=solar_data  OutDataTypeStr=double  SampleTime=0.01
  IGBT/Diode : spsIGBTDiodeLib/IGBT//Diode  Ron=1e-3  Rs=1e5  Cs=inf  Measurements=off
  L_boost : spsSeriesRLCBranchLib/Series RLC Branch  LConnTagsString=__new0  RConnTagsString=__new0  BranchType=L  Resistance=1e-3  Inductance=73e-3  SetiL0=off  InitialCurrent=0  Capacitance=100e-6  Setx0=off  InitialVoltage=230  Measurements=None
  MPPT : Subsystem
  PV Array1 : spsPVArrayLib/PV Array  Npar=5  Nser=2  PlotType=array @ 1000 W/m2 & specified temperatures  S_vec="[ 1000  500  100 ]"  Temp_C_vec="[ 45 25  ]"  ModuleName=SunPower SPR-415E-WHT-D  PlotWhenSelected=off  Pm=414.801  Ncell=128  Voc=85.3  Isc=6.09  Vm=72.9  Im=5.69  beta_Voc_pc=-0.229  alpha_Isc_pc=0.030706  beta_Voc=-0.19534  alpha_Isc=0.00187  IL=6.0978  I0=7.1698e-13  nI=0.87223  Rsh=419.7781  Rs=0.53711  RobustModel=off  RobustCellTemperature=313.3991  BAL=on  Tc=1e-6  Tfilter=5e-5
  RC_out : spsParallelRLCBranchLib/Parallel RLC Branch  LConnTagsString=a  RConnTagsString=__new0  BranchType=C  Resistance=5  Inductance=1e-3  SetiL0=off  InitialCurrent=0  Capacitance=5*768e-6  Setx0=off  InitialVoltage=700  Measurements=None
  Two-Level Converter : spsTwoLevelConverterLib/Two-Level Converter  ModelType=Switching devices  Ron=1e-3  Rs=1e6  Cs=inf  Vforward=[0,0]  Ron_Diode=1e-3  Rs_Diode=1e6  Cs_Diode=inf  Vf_Diode=1e-3  Rs_CurrentSource=inf  Ron_ACsource=1e-3
  Voltage Measurement : spsVoltageMeasurementLib/Voltage Measurement  PhasorSimulation=off  OutputType=Complex  PSBequivalent=0
  A : PMIOPort  Side=Left
  B : PMIOPort  Port=2  Side=Left
  C : PMIOPort  Port=3  Side=Left
  tag scope: Vdc_meas_6=global, i_pv_6=global, irr_6=global, v_pv_6=global
  wires:
  Voltage Measurement/1 -> [Vdc_meas_6]
  BL/1 -> Two-Level Converter/2
  Bus Selector1/3 -> [irr_6]  "<Irradiance (W/m2)>"
  Bus Selector1/1 -> [v_pv_6]  "<V_PV>"
  Constant4/1 -> PV Array1/2
  "  "/1 -> Two-Level Converter/1
  Bus Selector1/2 -> [i_pv_6]  "<I_PV>"
  PV Array1/1 -> Bus Selector1/1
  MPPT/1(P) -> IGBT/Diode/1
  From Workspace2/1 -> PV Array1/1
  connections:
  A/RConn1 -- Two-Level Converter/LConn1
  Two-Level Converter/RConn2 -- RC_out/RConn1 -- Voltage Measurement/LConn2 -- IGBT/Diode/RConn1 -- C_in/RConn1 -- PV Array1/RConn2
  Diode/LConn1 -- IGBT/Diode/LConn1 -- L_boost/RConn1
  C_in/LConn1 -- PV Array1/RConn1 -- L_boost/LConn1
  RC_out/LConn1 -- Diode/RConn1 -- Voltage Measurement/LConn1 -- Two-Level Converter/RConn1
  C/RConn1 -- Two-Level Converter/LConn3
  B/RConn1 -- Two-Level Converter/LConn2

== system Integration/Subsystem19 ==
  Ground1 : spsGroundLib/Ground  LConnTagsString=a
  Subsystem2 : Subsystem
  load : Scope  NumInputPorts=4
  A : PMIOPort  Side=Left
  B : PMIOPort  Port=2  Side=Left
  C : PMIOPort  Port=3  Side=Left
  wires:
  Subsystem2/4(Q_load) -> load/4
  Subsystem2/2(I_load) -> load/2
  Subsystem2/3(P_load) -> load/3
  Subsystem2/1(V_load) -> load/1
  connections:
  Subsystem2/LConn2 -- B/RConn1
  Subsystem2/LConn4 -- Ground1/LConn1
  Subsystem2/LConn1 -- A/RConn1
  Subsystem2/LConn3 -- C/RConn1

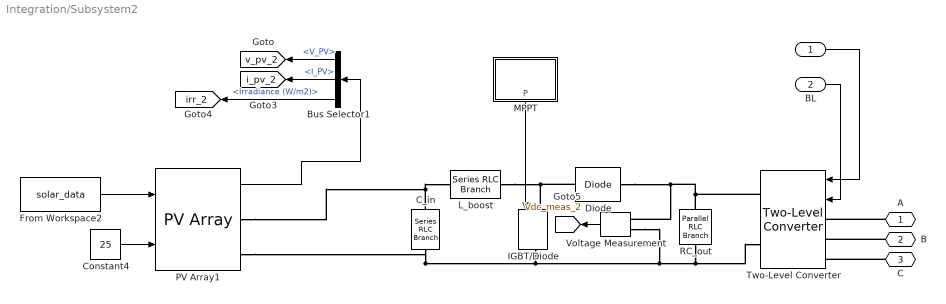
== system Integration/Subsystem2 ==
  "  " : Inport
  BL : Inport  Port=2
  Bus Selector1 : BusSelector  OutputSignals=V_PV,I_PV,Irradiance (W/m2)
  C_in : spsSeriesRLCBranchLib/Series RLC Branch  LConnTagsString=__new0  RConnTagsString=__new0  BranchType=C  Resistance=1e-5  Inductance=1e-3  SetiL0=off  InitialCurrent=0  Capacitance=3029e-6  Setx0=off  InitialVoltage=426.5  Measurements=Branch voltage and current
  Constant4 : Constant  Value=25
  Diode : spsDiodeLib/Diode  Ron=0.001  Lon=0  Vf=0.8  IC=0  UseSnubber=0  Rs=500  Cs=250e-9  Measurements=off
  From Workspace2 : FromWorkspace  VariableName=solar_data  OutDataTypeStr=double  SampleTime=0.01
  IGBT/Diode : spsIGBTDiodeLib/IGBT//Diode  Ron=1e-3  Rs=1e5  Cs=inf  Measurements=off
  L_boost : spsSeriesRLCBranchLib/Series RLC Branch  LConnTagsString=__new0  RConnTagsString=__new0  BranchType=L  Resistance=1e-3  Inductance=60e-3  SetiL0=off  InitialCurrent=0  Capacitance=100e-6  Setx0=off  InitialVoltage=230  Measurements=None
  MPPT : Subsystem
  PV Array1 : spsPVArrayLib/PV Array  Npar=2  Nser=6  PlotType=array @ 1000 W/m2 & specified temperatures  S_vec="[ 1000  500  100 ]"  Temp_C_vec="[ 45 25  ]"  ModuleName=SunPower SPR-415E-WHT-D  PlotWhenSelected=off  Pm=414.801  Ncell=128  Voc=85.3  Isc=6.09  Vm=72.9  Im=5.69  beta_Voc_pc=-0.229  alpha_Isc_pc=0.030706  beta_Voc=-0.19534  alpha_Isc=0.00187  IL=6.0978  I0=7.1698e-13  nI=0.87223  Rsh=419.7781  Rs=0.53711  RobustModel=off  RobustCellTemperature=313.3991  BAL=on  Tc=1e-6  Tfilter=5e-5
  RC_out : spsParallelRLCBranchLib/Parallel RLC Branch  LConnTagsString=a  RConnTagsString=__new0  BranchType=C  Resistance=5  Inductance=1e-3  SetiL0=off  InitialCurrent=0  Capacitance=5*922e-6  Setx0=off  InitialVoltage=700  Measurements=None
  Two-Level Converter : spsTwoLevelConverterLib/Two-Level Converter  ModelType=Switching devices  Ron=1e-3  Rs=1e6  Cs=inf  Vforward=[0,0]  Ron_Diode=1e-3  Rs_Diode=1e6  Cs_Diode=inf  Vf_Diode=1e-3  Rs_CurrentSource=inf  Ron_ACsource=1e-3
  Voltage Measurement : spsVoltageMeasurementLib/Voltage Measurement  PhasorSimulation=off  OutputType=Complex  PSBequivalent=0
  A : PMIOPort  Side=Left
  B : PMIOPort  Port=2  Side=Left
  C : PMIOPort  Port=3  Side=Left
  tag scope: Vdc_meas_2=global, i_pv_2=global, irr_2=global, v_pv_2=global
  wires:
  Voltage Measurement/1 -> [Vdc_meas_2]
  BL/1 -> Two-Level Converter/2
  Bus Selector1/3 -> [irr_2]  "<Irradiance (W/m2)>"
  Bus Selector1/1 -> [v_pv_2]  "<V_PV>"
  Constant4/1 -> PV Array1/2
  "  "/1 -> Two-Level Converter/1
  Bus Selector1/2 -> [i_pv_2]  "<I_PV>"
  PV Array1/1 -> Bus Selector1/1
  MPPT/1(P) -> IGBT/Diode/1
  From Workspace2/1 -> PV Array1/1
  connections:
  A/RConn1 -- Two-Level Converter/LConn1
  Two-Level Converter/RConn2 -- RC_out/RConn1 -- Voltage Measurement/LConn2 -- IGBT/Diode/RConn1 -- C_in/RConn1 -- PV Array1/RConn2
  Diode/LConn1 -- IGBT/Diode/LConn1 -- L_boost/RConn1
  C_in/LConn1 -- PV Array1/RConn1 -- L_boost/LConn1
  RC_out/LConn1 -- Two-Level Converter/RConn1 -- Diode/RConn1 -- Voltage Measurement/LConn1
  C/RConn1 -- Two-Level Converter/LConn3
  B/RConn1 -- Two-Level Converter/LConn2

== system Integration/Subsystem3 ==
  Series RLC Branch1 : spsSeriesRLCBranchLib/Series RLC Branch  LConnTagsString=__new0  RConnTagsString=__new0  BranchType=RC  Resistance=10  Inductance=1e-3  SetiL0=off  InitialCurrent=0  Capacitance=3*15e-6  Setx0=off  InitialVoltage=0  Measurements=None
  Series RLC Branch2 : spsSeriesRLCBranchLib/Series RLC Branch  LConnTagsString=__new0  RConnTagsString=__new0  BranchType=RC  Resistance=10  Inductance=1e-3  SetiL0=off  InitialCurrent=0  Capacitance=3*15e-6  Setx0=off  InitialVoltage=0  Measurements=None
  Series RLC Branch3 : spsSeriesRLCBranchLib/Series RLC Branch  LConnTagsString=__new0  RConnTagsString=__new0  BranchType=RC  Resistance=10  Inductance=1e-3  SetiL0=off  InitialCurrent=0  Capacitance=3*15e-6  Setx0=off  InitialVoltage=0  Measurements=None
  Three-Phase Series RLC Branch1 : spsThreePhaseSeriesRLCBranchLib/Three-Phase Series RLC Branch  LConnTagsString=A|B|C  RConnTagsString=A|B|C  BranchType=L  Resistance=1  Inductance=3*6e-3  Capacitance=1e-6  Measurements=None
  Three-Phase Breaker : spsThreePhaseBreakerLib/Three-Phase Breaker  InitialState=closed  SwitchA=on  SwitchB=on  SwitchC=on  SwitchTimes="[1/60  5/60]"  External=off  BreakerResistance=0.01  SnubberResistance=1e6  SnubberCapacitance=inf  Measurements=None
  A : PMIOPort  Side=Left
  B : PMIOPort  Port=2  Side=Left
  C : PMIOPort  Port=3  Side=Left
  a : PMIOPort  Port=4  Side=Right
  b : PMIOPort  Port=5  Side=Right
  c : PMIOPort  Port=6  Side=Right
  connections:
  Series RLC Branch1/LConn1 -- Three-Phase Series RLC Branch1/RConn2 -- Three-Phase Breaker/LConn2 -- Series RLC Branch3/RConn1
  Series RLC Branch1/RConn1 -- Three-Phase Breaker/LConn3 -- Three-Phase Series RLC Branch1/RConn3 -- Series RLC Branch2/RConn1
  Series RLC Branch3/LConn1 -- Three-Phase Series RLC Branch1/RConn1 -- Three-Phase Breaker/LConn1 -- Series RLC Branch2/LConn1
  Three-Phase Series RLC Branch1/LConn1 -- A/RConn1
  Three-Phase Series RLC Branch1/LConn2 -- B/RConn1
  Three-Phase Series RLC Branch1/LConn3 -- C/RConn1
  Three-Phase Breaker/RConn1 -- a/RConn1
  b/RConn1 -- Three-Phase Breaker/RConn2
  c/RConn1 -- Three-Phase Breaker/RConn3

== system Integration/Subsystem4 ==
  Ground1 : spsGroundLib/Ground  LConnTagsString=a
  Subsystem2 : Subsystem
  load : Scope  NumInputPorts=4
  A : PMIOPort  Side=Left
  B : PMIOPort  Port=2  Side=Left
  C : PMIOPort  Port=3  Side=Left
  wires:
  Subsystem2/4(Q_load) -> load/4
  Subsystem2/2(I_load) -> load/2
  Subsystem2/3(P_load) -> load/3
  Subsystem2/1(V_load) -> load/1
  connections:
  Subsystem2/LConn2 -- B/RConn1
  Subsystem2/LConn4 -- Ground1/LConn1
  Subsystem2/LConn1 -- A/RConn1
  Subsystem2/LConn3 -- C/RConn1

== system Integration/Subsystem5 ==
  Ground : spsGroundLib/Ground  LConnTagsString=a
  "Grounding Transformer " : spsGroundingTransformerLib/Grounding Transformer   UNITS=SI  NominalPower="[3e3   50]"  NominalVoltage=0.4e3  ZeroSequenceImpedance_pu=[0.025 0.75]  MagnetizationBranch_pu=[500 500]  ZeroSequenceImpedance_SI=[1.3333 40]  MagnetizationBranch_SI=[26667 26667]  Measurements=All voltages and currents
      settings: LibrarySourceBlock=|
      | sps_lib/Power Grid Elements/Grounding
      | Transformer
  Three-Phase Series RLC Branch1 : spsThreePhaseSeriesRLCBranchLib/Three-Phase Series RLC Branch  LConnTagsString=A|B|C  RConnTagsString=A|B|C  BranchType=RL  Resistance=0.02  Inductance=3e-3  Capacitance=1e-6  Measurements=None
  Three-Phase Source : spsThreePhaseSourceLib/Three-Phase Source  InternalConnection=Yg  VoltagePhases=off  Voltage=400  PhaseAngle=0  Voltage_phases=[25e3 25e3 25e3]/sqrt(3)  PhaseAngles_phases=[0 -120 +120]  Frequency=50  NonIdealSource=on  SpecifyImpedance=on  Resistance=0.0113  Inductance=36e-6  ShortCircuitLevel=5e6  BaseVoltage=400  XRratio=2  BusType=swing  Pref=10e3  Qref=0  Prefabc=[10e3, 10e3, 10e3]  Qrefabc=[0, 0, 0]  Qmin=-inf  Qmax=inf
  A : PMIOPort  Side=Left
  B : PMIOPort  Port=2  Side=Left
  C : PMIOPort  Port=3  Side=Left
  connections:
  "Grounding Transformer "/RConn1 -- Ground/LConn1
  Three-Phase Series RLC Branch1/LConn3 -- Three-Phase Source/RConn3
  Three-Phase Series RLC Branch1/LConn2 -- Three-Phase Source/RConn2
  Three-Phase Series RLC Branch1/RConn1 -- A/RConn1 -- "Grounding Transformer "/LConn1
  Three-Phase Series RLC Branch1/LConn1 -- Three-Phase Source/RConn1
  Three-Phase Series RLC Branch1/RConn3 -- C/RConn1 -- "Grounding Transformer "/LConn3
  Three-Phase Series RLC Branch1/RConn2 -- B/RConn1 -- "Grounding Transformer "/LConn2

== system Integration/Subsystem6 ==
  Ground1 : spsGroundLib/Ground  LConnTagsString=a
  Subsystem2 : Subsystem
  load : Scope  NumInputPorts=4
  A : PMIOPort  Side=Left
  B : PMIOPort  Port=2  Side=Left
  C : PMIOPort  Port=3  Side=Left
  wires:
  Subsystem2/4(Q_load) -> load/4
  Subsystem2/2(I_load) -> load/2
  Subsystem2/3(P_load) -> load/3
  Subsystem2/1(V_load) -> load/1
  connections:
  Subsystem2/LConn2 -- B/RConn1
  Subsystem2/LConn4 -- Ground1/LConn1
  Subsystem2/LConn1 -- A/RConn1
  Subsystem2/LConn3 -- C/RConn1

== system Integration/Subsystem7 ==
  Ground1 : spsGroundLib/Ground  LConnTagsString=a
  Subsystem2 : Subsystem
  load : Scope  NumInputPorts=4
  A : PMIOPort  Side=Left
  B : PMIOPort  Port=2  Side=Left
  C : PMIOPort  Port=3  Side=Left
  wires:
  Subsystem2/4(Q_load) -> load/4
  Subsystem2/2(I_load) -> load/2
  Subsystem2/3(P_load) -> load/3
  Subsystem2/1(V_load) -> load/1
  connections:
  Subsystem2/LConn2 -- B/RConn1
  Subsystem2/LConn4 -- Ground1/LConn1
  Subsystem2/LConn1 -- A/RConn1
  Subsystem2/LConn3 -- C/RConn1

== system Integration/Subsystem8 ==
  Series RLC Branch1 : spsSeriesRLCBranchLib/Series RLC Branch  LConnTagsString=__new0  RConnTagsString=__new0  BranchType=RC  Resistance=10  Inductance=1e-3  SetiL0=off  InitialCurrent=0  Capacitance=3*15e-6  Setx0=off  InitialVoltage=0  Measurements=None
  Series RLC Branch2 : spsSeriesRLCBranchLib/Series RLC Branch  LConnTagsString=__new0  RConnTagsString=__new0  BranchType=RC  Resistance=10  Inductance=1e-3  SetiL0=off  InitialCurrent=0  Capacitance=3*15e-6  Setx0=off  InitialVoltage=0  Measurements=None
  Series RLC Branch3 : spsSeriesRLCBranchLib/Series RLC Branch  LConnTagsString=__new0  RConnTagsString=__new0  BranchType=RC  Resistance=10  Inductance=1e-3  SetiL0=off  InitialCurrent=0  Capacitance=3*15e-6  Setx0=off  InitialVoltage=0  Measurements=None
  Three-Phase Series RLC Branch1 : spsThreePhaseSeriesRLCBranchLib/Three-Phase Series RLC Branch  LConnTagsString=A|B|C  RConnTagsString=A|B|C  BranchType=L  Resistance=1  Inductance=3*6e-3  Capacitance=1e-6  Measurements=None
  Three-Phase Breaker : spsThreePhaseBreakerLib/Three-Phase Breaker  InitialState=closed  SwitchA=on  SwitchB=on  SwitchC=on  SwitchTimes="[1/60  5/60]"  External=off  BreakerResistance=0.01  SnubberResistance=1e6  SnubberCapacitance=inf  Measurements=None
  A : PMIOPort  Side=Left
  B : PMIOPort  Port=2  Side=Left
  C : PMIOPort  Port=3  Side=Left
  a : PMIOPort  Port=4  Side=Right
  b : PMIOPort  Port=5  Side=Right
  c : PMIOPort  Port=6  Side=Right
  connections:
  Series RLC Branch1/LConn1 -- Three-Phase Series RLC Branch1/RConn2 -- Three-Phase Breaker/LConn2 -- Series RLC Branch3/RConn1
  Series RLC Branch1/RConn1 -- Three-Phase Breaker/LConn3 -- Three-Phase Series RLC Branch1/RConn3 -- Series RLC Branch2/RConn1
  Series RLC Branch3/LConn1 -- Three-Phase Series RLC Branch1/RConn1 -- Three-Phase Breaker/LConn1 -- Series RLC Branch2/LConn1
  Three-Phase Series RLC Branch1/LConn1 -- A/RConn1
  Three-Phase Series RLC Branch1/LConn2 -- B/RConn1
  Three-Phase Series RLC Branch1/LConn3 -- C/RConn1
  Three-Phase Breaker/RConn1 -- a/RConn1
  b/RConn1 -- Three-Phase Breaker/RConn2
  c/RConn1 -- Three-Phase Breaker/RConn3

== system Integration/Subsystem9 ==
  "  " : Inport
  BL : Inport  Port=2
  Bus Selector1 : BusSelector  OutputSignals=V_PV,I_PV,Irradiance (W/m2)
  C_in : spsSeriesRLCBranchLib/Series RLC Branch  LConnTagsString=__new0  RConnTagsString=__new0  BranchType=C  Resistance=1e-5  Inductance=1e-3  SetiL0=off  InitialCurrent=0  Capacitance=314e-6  Setx0=off  InitialVoltage=426.5  Measurements=Branch voltage and current
  Constant4 : Constant  Value=25
  Diode : spsDiodeLib/Diode  Ron=0.001  Lon=0  Vf=0.8  IC=0  UseSnubber=0  Rs=500  Cs=250e-9  Measurements=off
  From Workspace2 : FromWorkspace  VariableName=solar_data  OutDataTypeStr=double  SampleTime=0.01
  IGBT/Diode : spsIGBTDiodeLib/IGBT//Diode  Ron=1e-3  Rs=1e5  Cs=inf  Measurements=off
  L_boost : spsSeriesRLCBranchLib/Series RLC Branch  LConnTagsString=__new0  RConnTagsString=__new0  BranchType=L  Resistance=1e-3  Inductance=157e-3  SetiL0=off  InitialCurrent=0  Capacitance=100e-6  Setx0=off  InitialVoltage=230  Measurements=None
  MPPT : Subsystem
  PV Array1 : spsPVArrayLib/PV Array  Npar=3  Nser=5  PlotType=array @ 1000 W/m2 & specified temperatures  S_vec="[ 1000  500  100 ]"  Temp_C_vec="[ 45 25  ]"  ModuleName=SunPower SPR-415E-WHT-D  PlotWhenSelected=off  Pm=414.801  Ncell=128  Voc=85.3  Isc=6.09  Vm=72.9  Im=5.69  beta_Voc_pc=-0.229  alpha_Isc_pc=0.030706  beta_Voc=-0.19534  alpha_Isc=0.00187  IL=6.0978  I0=7.1698e-13  nI=0.87223  Rsh=419.7781  Rs=0.53711  RobustModel=off  RobustCellTemperature=313.3991  BAL=on  Tc=1e-6  Tfilter=5e-5
  RC_out : spsParallelRLCBranchLib/Parallel RLC Branch  LConnTagsString=a  RConnTagsString=__new0  BranchType=C  Resistance=5  Inductance=1e-3  SetiL0=off  InitialCurrent=0  Capacitance=5*239e-6  Setx0=off  InitialVoltage=700  Measurements=None
  Two-Level Converter : spsTwoLevelConverterLib/Two-Level Converter  ModelType=Switching devices  Ron=1e-3  Rs=1e6  Cs=inf  Vforward=[0,0]  Ron_Diode=1e-3  Rs_Diode=1e6  Cs_Diode=inf  Vf_Diode=1e-3  Rs_CurrentSource=inf  Ron_ACsource=1e-3
  Voltage Measurement : spsVoltageMeasurementLib/Voltage Measurement  PhasorSimulation=off  OutputType=Complex  PSBequivalent=0
  A : PMIOPort  Side=Left
  B : PMIOPort  Port=2  Side=Left
  C : PMIOPort  Port=3  Side=Left
  tag scope: Vdc_meas_3=global, i_pv_3=global, irr_3=global, v_pv_3=global
  wires:
  Voltage Measurement/1 -> [Vdc_meas_3]
  BL/1 -> Two-Level Converter/2
  Bus Selector1/3 -> [irr_3]  "<Irradiance (W/m2)>"
  Bus Selector1/1 -> [v_pv_3]  "<V_PV>"
  Constant4/1 -> PV Array1/2
  "  "/1 -> Two-Level Converter/1
  Bus Selector1/2 -> [i_pv_3]  "<I_PV>"
  PV Array1/1 -> Bus Selector1/1
  MPPT/1(P) -> IGBT/Diode/1
  From Workspace2/1 -> PV Array1/1
  connections:
  A/RConn1 -- Two-Level Converter/LConn1
  Two-Level Converter/RConn2 -- RC_out/RConn1 -- Voltage Measurement/LConn2 -- IGBT/Diode/RConn1 -- C_in/RConn1 -- PV Array1/RConn2
  Diode/LConn1 -- IGBT/Diode/LConn1 -- L_boost/RConn1
  C_in/LConn1 -- PV Array1/RConn1 -- L_boost/LConn1
  RC_out/LConn1 -- Two-Level Converter/RConn1 -- Diode/RConn1 -- Voltage Measurement/LConn1
  C/RConn1 -- Two-Level Converter/LConn3
  B/RConn1 -- Two-Level Converter/LConn2

== system Integration/VSC Control ==
  note: VSC Main Controller
  V : Inport  PortDimensions=3
  I : Inport  Port=2  PortDimensions=3
  Vdc : Inport  Port=3  PortDimensions=1
  Current Regulator : Subsystem
  Iq_ref : Constant  Value=0
  Mux : Mux  Inputs=2
  PLL & Measurements : Subsystem
  PWM Generator (2-Level) : spsPWMGenerator2LevelLib/PWM Generator (2-Level)  ModulatorType=Three-phase bridge (6 pulses)  ModulatorMode=Unsynchronized  Fc=27*50*8  Pc=90  nF=27  MinMax="[ -1  1 ]"  SamplingTechnique=Natural  ModulatingSignals=off  m=0.8  Freq=60  Phase=0  Ts=Ts_Control  ShowCarrierOutport=off
  Product : Product
  Ramp : simulink/Sources/Ramp  slope=1/0.02  start=0  InitialOutput=0
  Saturation : Saturate  UpperLimit=1  LowerLimit=0
  Scope : Scope  NumInputPorts=2
  Uabc_ref Generation max (m) = 1 : Subsystem
  Unit Delay : UnitDelay  SampleTime=Ts_Control  HasFrameUpgradeWarning=on
  VDC Regulator : Subsystem
  Vdc_ref1 : Constant  Value=Vdc_ref
  Uref : Outport  VectorParamsAs1DForOutWhenUnconnected=off
  wires:
  Vdc_ref1/1 -> VDC Regulator/2(Vdc_ref)
  Uabc_ref Generation max (m) = 1/1(Uabc_ref) -> Unit Delay/1
  Unit Delay/1 -> PWM Generator (2-Level)/1
  I/1 -> PLL & Measurements/2(Iabc_prim)
  V/1 -> PLL & Measurements/1(Vabc_prim)
  Vdc/1 -> VDC Regulator/1(Vdc_meas)
  PLL & Measurements/2(VdVq_prim) -> Current Regulator/1(VdVq_meas)
  PLL & Measurements/3(IdIq_prim) -> Current Regulator/2(IdIq_meas)
  Mux/1 -> Current Regulator/3(IdIq_ref)
  Iq_ref/1 -> Mux/2
  PLL & Measurements/1(wt) -> Uabc_ref Generation max (m) = 1/1(wt)
  VDC Regulator/1(Id_ref) -> Mux/1
  PWM Generator (2-Level)/1 -> Product/1
  Current Regulator/1(VdVq_conv) -> Scope/2, Uabc_ref Generation max (m) = 1/2(VdVq_conv)
  Product/1 -> Scope/1, Uref/1
  Ramp/1 -> Saturation/1
  Saturation/1 -> Product/2
